simulink model "UUV_inv_dyn"  (R2020a)
settings: Solver=VariableStepAuto  StartTime=0.0  StopTime=10.0  RelTol=1e-3
settings Model: Creator=Sebas  LastModifiedBy=Sebas

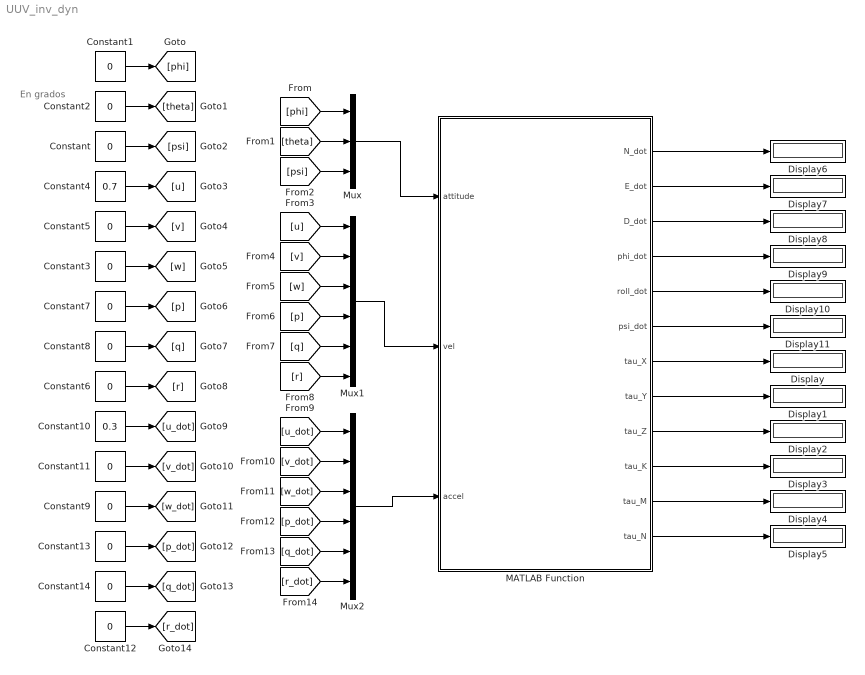
== system UUV_inv_dyn ==
  note: En grados
  Constant{,1..3,5..9,11..14} (13 alike) : Constant  Value=0
  Constant10 : Constant  Value=0.3
  Constant4 : Constant  Value=0.7
  Display{,1..11} (12 alike) : Display
  MATLAB Function : MATLAB Function  TreatAsAtomicUnit=on
  Mux : Mux  Inputs=3
  Mux1 : Mux  Inputs=6
  Mux2 : Mux  Inputs=6
  wires:
  MATLAB Function/7(tau_X) -> Display/1
  Mux/1 -> MATLAB Function/1(attitude)
  Mux1/1 -> MATLAB Function/2(vel)
  Mux2/1 -> MATLAB Function/3(accel)
  Constant1/1 -> [phi]
  Constant2/1 -> [theta]
  Constant/1 -> [psi]
  Constant4/1 -> [u]
  Constant5/1 -> [v]
  Constant3/1 -> [w]
  Constant9/1 -> [w_dot]
  Constant6/1 -> [r]
  Constant10/1 -> [u_dot]
  Constant8/1 -> [q]
  Constant7/1 -> [p]
  Constant11/1 -> [v_dot]
  Constant13/1 -> [p_dot]
  Constant14/1 -> [q_dot]
  Constant12/1 -> [r_dot]
  [phi] -> Mux/1
  [theta] -> Mux/2
  [psi] -> Mux/3
  [v] -> Mux1/2
  [u] -> Mux1/1
  [w] -> Mux1/3
  [q] -> Mux1/5
  [p] -> Mux1/4
  [r] -> Mux1/6
  [u_dot] -> Mux2/1
  [v_dot] -> Mux2/2
  [r_dot] -> Mux2/6
  [q_dot] -> Mux2/5
  [p_dot] -> Mux2/4
  [w_dot] -> Mux2/3
  MATLAB Function/8(tau_Y) -> Display1/1
  MATLAB Function/9(tau_Z) -> Display2/1
  MATLAB Function/10(tau_K) -> Display3/1
  MATLAB Function/11(tau_M) -> Display4/1
  MATLAB Function/12(tau_N) -> Display5/1
  MATLAB Function/2(E_dot) -> Display7/1
  MATLAB Function/3(D_dot) -> Display8/1
  MATLAB Function/4(phi_dot) -> Display9/1
  MATLAB Function/5(roll_dot) -> Display10/1
  MATLAB Function/6(psi_dot) -> Display11/1
  MATLAB Function/1(N_dot) -> Display6/1

== matlab function UUV_inv_dyn/MATLAB Function ==
  data: N_dot output; E_dot output; D_dot output; phi_dot output; roll_dot output; psi_dot output; attitude input; tau_X output; vel input; accel input; tau_Y output; tau_Z output; tau_K output; tau_M output; tau_N output
function [N_dot,E_dot,D_dot,phi_dot,roll_dot,psi_dot,tau_X,tau_Y,tau_Z,tau_K,tau_M,tau_N]  = UUV_model(attitude, vel, accel)
% Skew symmetric matrix
S = @(s) [0    -s(3) s(2);
          s(3) 0     -s(1);
          -s(2) s(1)  0    ];  
      
% Parameters
m = 24;
vol = 0.02306187;
W = m*9.81;
B = W*1.005; %1000*9.81*vol;

r_g = [0 0 0].';    % Distance from origin to center of mass
r_b = [0 0 -0.10726].';    % Distance from origin to center of buoyancy
I_g = [0.900121387  -0.000186482 0.0072251;
       -0.000186482 1.754494427  0.020319615;
       0.0072251    0.020319615  1.43389     ];

phi = deg2rad(attitude(1)); % roll
theta = deg2rad(attitude(2)); % pitch
psi = deg2rad(attitude(3)); % yaw

% Linear damping coefficients
X_u = -0.3431;
Y_v = 0.0518;
Z_w = -0.5841;
K_p = 0.0064;
M_q = 0.04;
N_r = -0.1063;

% Cuadratic damping coefficients
X_uu = -111.7397;
Y_vv = -44.4058;
Z_ww = -157.1951;
K_pp = -0.4634;
M_qq = -0.2902;
N_rr = -2.2897;

%------------ UUV kinematics ----------------%
% Linear velocities
% For a zxy rotation sequence
N_dot = vel(1)*cos(psi)*cos(theta) + vel(2)*[cos(psi)*sin(theta)*sin(phi) - sin(psi)*cos(phi)] + vel(3)*[sin(psi)*sin(phi) + cos(psi)*cos(phi)*sin(theta)];

E_dot = vel(1)*sin(psi)*cos(theta) + vel(2)*[cos(psi)*cos(phi) + sin(phi)*sin(theta)*sin(psi)]+ vel(3)*[sin(theta)*sin(psi)*cos(phi) - cos(psi)*sin(phi)];

D_dot = -vel(1)*sin(theta) + vel(2)*cos(theta)*sin(phi) + vel(3)*cos(theta)*cos(phi);

%Angular velocities
phi_dot = vel(4) + vel(5)*sin(phi)*tan(theta) + vel(6)*cos(phi)*tan(theta);

roll_dot = vel(5)*cos(phi) - vel(6)*sin(phi);

psi_dot = vel(5)*(sin(phi)/cos(theta)) + vel(6)*(cos(phi)/cos(theta));

eta_dot = [N_dot, E_dot, D_dot, phi_dot, roll_dot, psi_dot];

%------------ UUV dynamic model parametrization ----------------%

% Rigid-Body Inertia Matrix
M_rb = [ m*eye(3)    -m*S(r_g);
         m*S(r_g)         I_g ];

% Added mass matrix
M_a = diag([16.8374 20.2748 35.3180 0.2165 0.6869 0.6157]);

% Mass matrix
M = M_rb + M_a;

% Rigid-body Coriolis-centripetal Matrix
C_rb = [ zeros(3)             -m*S(vel(1:3))-m*S(vel(4:6))*S(r_g);
        -m*S(vel(1:3))+m*S(r_g)*S(vel(4:6))            -S(I_g*vel(4:6))];

% Coreolis added mass matrix 
C_a = [ 0 0 0   0 -M_a(3,3)*vel(3) M_a(2,2)*vel(2) ;
        0 0 0   M_a(3,3)*vel(3) 0 -M_a(1,1)*vel(1) ;
        0 0 0  -M_a(2,2)*vel(2) M_a(1,1)*vel(1) 0  ;
        0 -M_a(3,3)*vel(3) M_a(2,2)*vel(2)  0 -M_a(6,6)*vel(6) M_a(5,5)*vel(5) ;
        M_a(3,3)*vel(3) 0 -M_a(1,1)*vel(1)  M_a(6,6)*vel(6) 0 -M_a(4,4)*vel(4) ;
       -M_a(2,2)*vel(2) M_a(1,1)*vel(1) 0   -M_a(5,5)*vel(5) M_a(4,4)*vel(4) 0  ];

% Coreolis matrix
C = C_rb + C_a;

% Restoring forces
g_eta = [ (W-B)*sin(theta);
          -(W-B)*cos(theta)*sin(phi);
          -(W-B)*cos(theta)*cos(phi);
          -(r_g(2)*W-r_b(2)*B)*cos(theta)*cos(phi) + (r_g(3)*W-r_b(3)*B)*cos(theta)*sin(phi);
           (r_g(3)*W-r_b(3)*B)*sin(theta)          + (r_g(1)*W-r_b(1)*B)*cos(theta)*cos(phi)
          -(r_g(1)*W-r_b(1)*B)*cos(theta)*sin(phi) - (r_g(2)*W-r_b(2)*B)*sin(theta)          ];
   
% Damping matrix
D_lin = -diag([X_u Y_v Z_w K_p M_q N_r]);
D_cuad = -diag([X_uu*abs(vel(1)) Y_vv*abs(vel(2)) Z_ww*abs(vel(3)) ...
               K_pp*abs(vel(4)) M_qq*abs(vel(5)) N_rr*abs(vel(6))]);
D = D_lin + D_cuad;

% Tau
tau = M*accel + C*vel + D*vel + g_eta;
tau_X = tau(1);
tau_Y = tau(2);
tau_Z = tau(3);
tau_K = tau(4);
tau_M = tau(5);
tau_N = tau(6);
